simulink model "Subsystem"  (R2019b)
settings: Solver=FixedStepAuto  StartTime=0.0  StopTime=testtime  RelTol=1e-3
InitFcn:
  | Discrete_Transfer_Fcn_Test_Parameters
StopFcn:
  | Verify_Discrete_Transfer_Fcn_Test_Filter
undefined symbols (not defined in the file): c1LPihc, c2LPihc, gainihc
settings Model: Creator=mblun  LastModifiedBy=cb50701
settings DataIOCC: SaveOutput=off  SaveTime=off
settings OptimizationCC: BlockReduction=off  ConditionallyExecuteInputs=off  DefaultParameterBehavior=Inlined
settings DebuggingCC: AlgebraicLoopMsg=error
settings HardwareCC: ProdBitPerPointer=32  ProdBitPerSizeT=32  ProdBitPerPtrDiffT=32  ProdLargestAtomicFloat=None  ProdIntDivRoundTo=Undefined  ProdEndianess=Unspecified  ProdWordSize=32  ProdHWDeviceType=ASIC/FPGA->ASIC/FPGA  TargetBitPerLong=64  TargetBitPerPointer=64  TargetBitPerSizeT=64  TargetBitPerPtrDiffT=64  TargetLongLongMode=on  TargetIntDivRoundTo=Zero  TargetEndianess=LittleEndian  TargetWordSize=64  TargetHWDeviceType=Custom Processor->MATLAB Host Computer  ProdEqTarget=off
settings SFSimCC: CustomCodeUndefinedFunction=UseInterfaceOnly

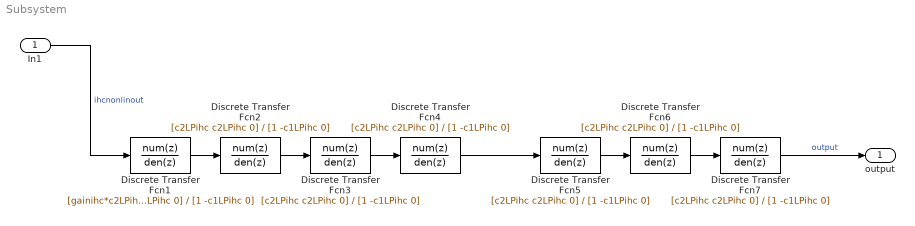
== system Subsystem ==
  In1 : Inport  OutDataTypeStr=single  PortDimensions=[1 1]  SampleTime=[2.0833333333333333e-05,0]
  Discrete Transfer Fcn1 : DiscreteTransferFcn  Numerator=[gainihc*c2LPihc gainihc*c2LPihc 0]  Denominator=[1 -c1LPihc 0]
  Discrete Transfer Fcn{2..7} (6 alike) : DiscreteTransferFcn  Numerator=[c2LPihc c2LPihc 0]  Denominator=[1 -c1LPihc 0]
  output : Outport  OutDataTypeStr=single  PortDimensions=[1 1]  SampleTime=[2.0833333333333333e-05,0]
  wires:
  Discrete Transfer Fcn1/1 -> Discrete Transfer Fcn2/1
  Discrete Transfer Fcn2/1 -> Discrete Transfer Fcn3/1
  Discrete Transfer Fcn3/1 -> Discrete Transfer Fcn4/1
  Discrete Transfer Fcn5/1 -> Discrete Transfer Fcn6/1
  In1/1 -> Discrete Transfer Fcn1/1  "ihcnonlinout"
  Discrete Transfer Fcn4/1 -> Discrete Transfer Fcn5/1
  Discrete Transfer Fcn7/1 -> output/1  "output"
  Discrete Transfer Fcn6/1 -> Discrete Transfer Fcn7/1
